simulink model "ex1_3sim"  (R2017a)
settings: Solver=VariableStepAuto  StartTime=0.0  StopTime=10.0  RelTol=1e-3
values from neighbouring files (symbols this model uses):
  A = [ -0.16 0 ; 0.16 -0.16]    [ex1_1.m]    (also in ex1_2.m = [-R/L -1/L; 1/C 0])
  B = [1/L; 0]    [ex1_2.m]
  X0 = [60; 0]    [ex1_1.m]    (also in ex1_2.m = [0; 0])
settings Model: Creator=erivelton  LastModifiedBy=erivelton

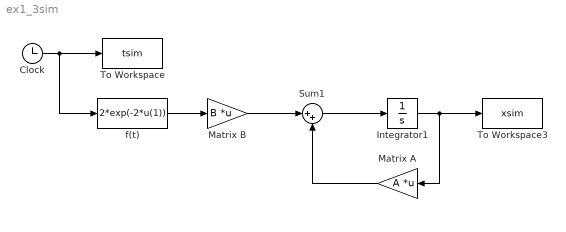
== system ex1_3sim ==
  Clock : Clock
  Integrator1 : Integrator  InitialCondition=X0
  Matrix A : Gain  Gain=A  Multiplication=Matrix(K*u)
  Matrix B : Gain  Gain=B  Multiplication=Matrix(K*u)
  Sum1 : Sum  Inputs=|++
  To Workspace : ToWorkspace  VariableName=tsim  SampleTime=-1
  To Workspace3 : ToWorkspace  VariableName=xsim  SampleTime=-1
  f(t) : MATLABFcn  MATLABFcn=2*exp(-2*u(1))
  wires:
  Integrator1/1 -> To Workspace3/1, Matrix A/1
  Matrix A/1 -> Sum1/2
  Matrix B/1 -> Sum1/1
  Sum1/1 -> Integrator1/1
  Clock/1 -> f(t)/1, To Workspace/1
  f(t)/1 -> Matrix B/1
